simulink model "Std_Treat"  (Simulink 7.5)
settings: Solver=ode45  StartTime=0.0  StopTime=10.0  RelTol=1e-3
undefined symbols (not defined in the file or in its folder): ctrller, scenario
settings Model: Creator=sriddle  LastModifiedBy=sriddle

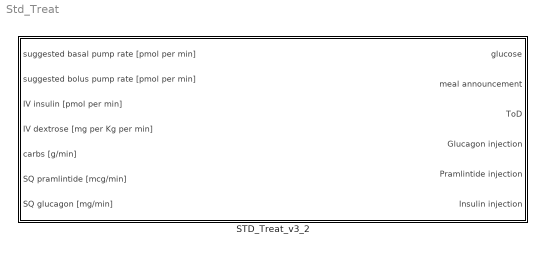
== system Std_Treat ==
  STD_Treat_v3_2 : Subsystem

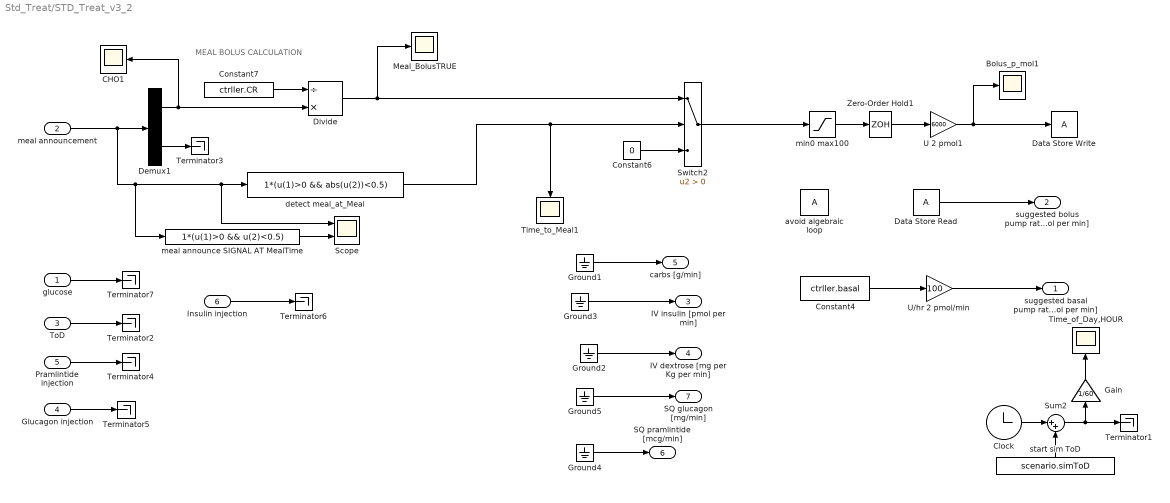
== system Std_Treat/STD_Treat_v3_2 ==
  note: MEAL BOLUS CALCULATION
  glucose : Inport
  meal announcement : Inport  Port=2
  ToD : Inport  Port=3
  Glucagon injection : Inport  Port=4
  Pramlintide injection : Inport  Port=5
  Insulin injection : Inport  Port=6
  Bolus_p_mol1 : Scope
      settings: YMin=0  YMax=60000  SaveName=ScopeData5
  CHO1 : Scope
      settings: YMin=0  YMax=60  SaveName=ScopeData15
  Clock : Clock
      settings: Decimation=10
  Constant4 : Constant  Value=ctrller.basal
  Constant6 : Constant  Value=0
  Constant7 : Constant  Value=ctrller.CR
  Data Store Read : DataStoreRead  DataStoreName=A  SampleTime=0
  Data Store Write : DataStoreWrite  DataStoreName=A  SampleTime=-1
  Demux1 : Demux  Outputs=2
  Divide : Product  Inputs=/*
  Gain : Gain  Gain=1/60
  Ground{1..5} (5 alike) : Ground
  Meal_BolusTRUE : Scope
      settings: YMin=0  SaveName=ScopeData20
  Scope : Scope  NumInputPorts=2
      settings: YMin=-5~-5  YMax=5~5  SaveName=ScopeData21
  Sum2 : Sum  Inputs=|++
  Switch2 : Switch  Criteria=u2 > Threshold
  Terminator{1..7} (7 alike) : Terminator
  Time_of_Day,HOUR : Scope
      settings: YMin=0  YMax=60000  SaveName=ScopeData22
  Time_to_Meal1 : Scope
      settings: SaveName=ScopeData23
  U 2 pmol1 : Gain  Gain=6000
  U/hr 2 pmol/min : Gain  Gain=100
  Zero-Order Hold1 : ZeroOrderHold
  avoid algebraic loop : DataStoreMemory  DataStoreName=A  ReadBeforeWriteMsg=warning  WriteAfterWriteMsg=warning  WriteAfterReadMsg=warning
  detect meal_at_Meal : Fcn  Expr=1*(u(1)>0 && abs(u(2))<0.5)
  meal announce SIGNAL AT MealTime : Fcn  Expr=1*(u(1)>0 && u(2)<0.5)  SampleTime=1
  min0 max100 : Saturate  UpperLimit=100  LowerLimit=0
  start sim ToD : Constant  Value=scenario.simToD
  suggested basal pump rate [pmol per min] : Outport
  suggested bolus pump rate [pmol per min] : Outport  Port=2
  IV insulin [pmol per min] : Outport  Port=3
  IV dextrose [mg per Kg per min] : Outport  Port=4
  carbs [g/min] : Outport  Port=5
  SQ pramlintide [mcg/min] : Outport  Port=6
  SQ glucagon [mg/min] : Outport  Port=7
  wires:
  Data Store Read/1 -> suggested bolus pump rate [pmol per min]/1
  U/hr 2 pmol/min/1 -> suggested basal pump rate [pmol per min]/1
  Constant4/1 -> U/hr 2 pmol/min/1
  ToD/1 -> Terminator2/1
  Constant6/1 -> Switch2/3
  detect meal_at_Meal/1 -> Switch2/2, Time_to_Meal1/1
  Constant7/1 -> Divide/1
  Demux1/1 -> Divide/2, CHO1/1
  meal announcement/1 -> Demux1/1, meal announce SIGNAL AT MealTime/1, detect meal_at_Meal/1, Scope/1
  Demux1/2 -> Terminator3/1
  Divide/1 -> Meal_BolusTRUE/1, Switch2/1
  Zero-Order Hold1/1 -> U 2 pmol1/1
  U 2 pmol1/1 -> Data Store Write/1, Bolus_p_mol1/1
  min0 max100/1 -> Zero-Order Hold1/1
  Clock/1 -> Sum2/1
  Sum2/1 -> Terminator1/1, Gain/1
  start sim ToD/1 -> Sum2/2
  Gain/1 -> Time_of_Day,HOUR/1
  Ground5/1 -> SQ glucagon [mg/min]/1
  Ground4/1 -> SQ pramlintide [mcg/min]/1
  Pramlintide injection/1 -> Terminator4/1
  Ground2/1 -> IV dextrose [mg per Kg per min]/1
  Glucagon injection/1 -> Terminator5/1
  Ground1/1 -> carbs [g/min]/1
  Ground3/1 -> IV insulin [pmol per min]/1
  meal announce SIGNAL AT MealTime/1 -> Scope/2
  Insulin injection/1 -> Terminator6/1
  glucose/1 -> Terminator7/1
  Switch2/1 -> min0 max100/1
